simulink model "roller_coaster_simulink"  (R2024a)
settings: Solver=VariableStepAuto  StartTime=0.0  StopTime=200  RelTol=1e-3
settings Model: Creator=bkpou  LastModifiedBy=bkpou

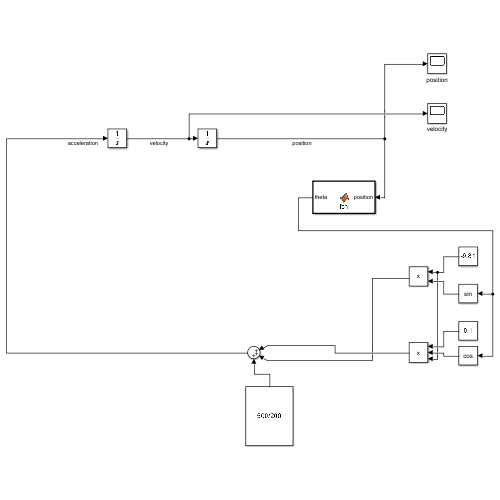
[thumbnail: Simulink's stored preview of the top-level diagram]
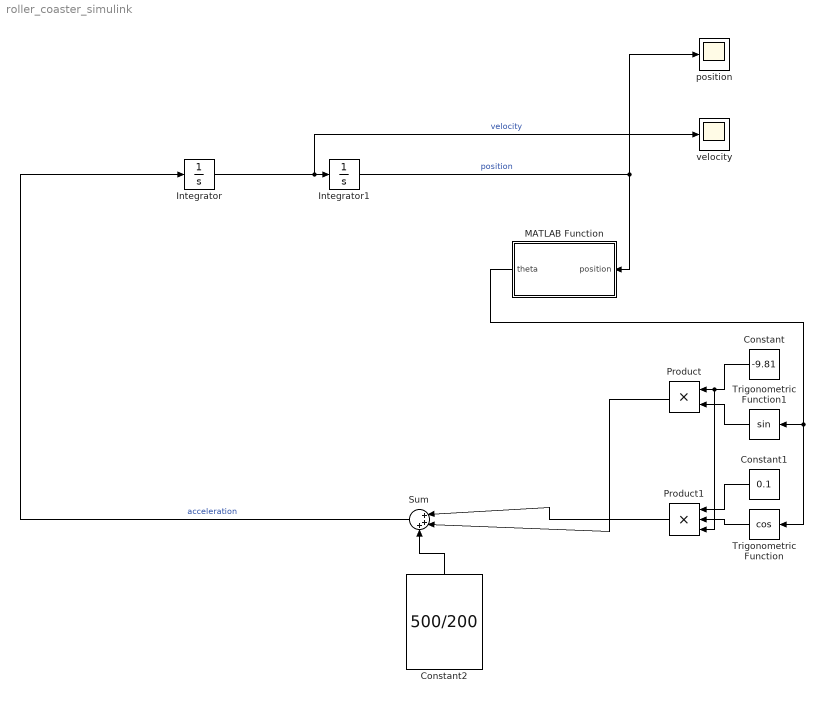
== system roller_coaster_simulink ==
  Constant : Constant  Value=-9.81
  Constant1 : Constant  Value=0.1
  Constant2 : Constant  Value=500/200
  Integrator : Integrator
  Integrator1 : Integrator
  MATLAB Function : MATLAB Function  TreatAsAtomicUnit=on
  Product : Product
  Product1 : Product  Inputs=3
  Sum : Sum  Inputs=|+++
  Trigonometric Function : Trigonometry  Operator=cos
  Trigonometric Function1 : Trigonometry
  position : Scope
  velocity : Scope
  wires:
  Integrator/1 -> velocity/1, Integrator1/1  "velocity"
  Sum/1 -> Integrator/1  "acceleration"
  Integrator1/1 -> position/1, MATLAB Function/1(position)  "position"
  Constant/1 -> Product1/3, Product/1
  Trigonometric Function1/1 -> Product/2
  MATLAB Function/1(theta) -> Trigonometric Function/1, Trigonometric Function1/1
  Constant1/1 -> Product1/1
  Trigonometric Function/1 -> Product1/2
  Product1/1 -> Sum/1
  Product/1 -> Sum/2
  Constant2/1 -> Sum/3

== matlab function roller_coaster_simulink/MATLAB Function ==
  data: position input; theta output
function theta = fcn(position)
    if position <= 10
        theta = 0;
    elseif position <= (10 + 10*cos(30))
        theta = 0.5236;
    else
        theta = 0;
   end
end
